simulink model "mod3_2plus1MASH_v2"  (Simulink 8.1)
settings: Solver=FixedStepDiscrete  StartTime=0.0  StopTime=80e-3  RelTol=1e-3
undefined symbols (not defined in the file): dfilt, Fs, modctrl
libraries: dspsigops x4, dspsrcs4 x2, dsparch4 x1
settings Model: Creator=amyles  LastModifiedBy=amyles
settings DataIOCC: MaxDataPoints=50000
settings OptimizationCC: InlineParams=on
settings DebuggingCC: StrictBusMsg=Warning
settings ModelReferenceCC: ModelReferenceNumInstancesAllowed=Single

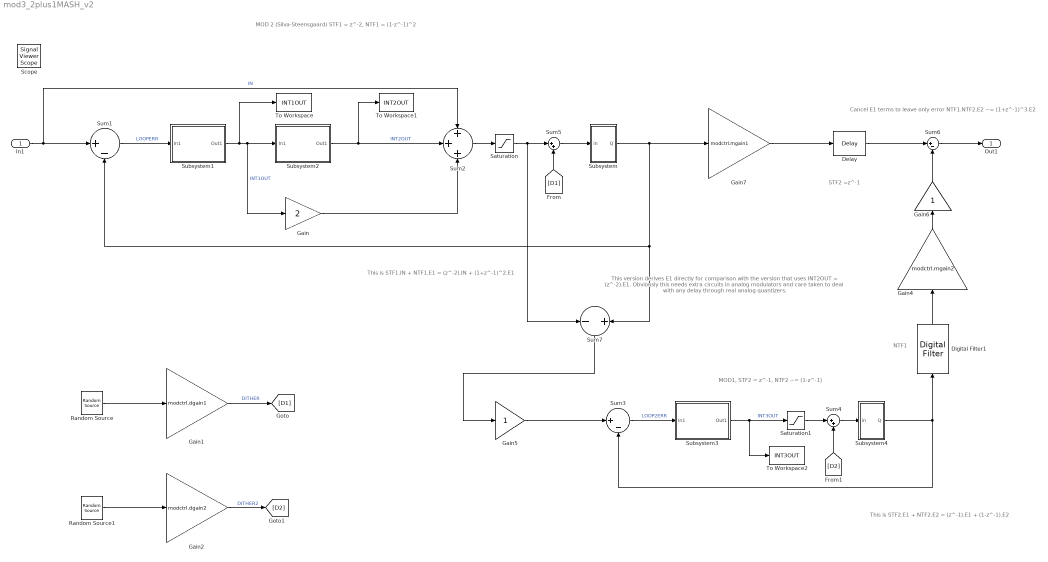
== system mod3_2plus1MASH_v2 ==
  note: MOD 2 (Silva-Steensgaard)
      | STF1 = z^-2, NTF1 = (1-z^-1)^2
  note: MOD1, STF2 = z^-1, NTF2 ~= (1-z^-1)
  note: This is STF2.E1 + NTF2.E2
      | = (z^-1).E1 + (1-z^-1).E2
  note: STF2
      | =z^-1
  note: NTF1
  note: Cancel E1 terms to leave
      | only error NTF1.NTF2.E2
      | ~= (1+z^-1)^3.E2
  note: This version derives E1
      | directly for comparison
      | with the version that uses
      | INT2OUT = (z^-2).E1.
      | Obviously this needs extra
      | circuits in analog modulators
      | and care taken to deal with
      | any delay through real
      | analog quantizers.
  note: This is STF1.IN + NTF1.E1
      | = (z^-2).IN + (1+z^-1)^2.E1
  In1 : Inport
  Delay : dspsigops/Delay  InputProcessing=Inherited (this choice will be removed - see release notes)  dly_unit=Samples  delay=1  ic_detail=off  dif_ic_for_ch=off  dif_ic_for_dly=off  ic=0  reset_popup=None
  Digital Filter1 : dsparch4/Digital Filter  TypePopup=FIR (all zeros)  IIRFiltStruct=Direct form II transposed  AllPoleFiltStruct=Direct form  FIRFiltStruct=Direct form  CoeffSource=Specify via dialog  NumCoeffs=[1 -2 1]  DenCoeffs=[1 0.1]  BiQuadCoeffs=[1 0.3 0.4 1 0.1 0.2]  LatticeCoeffs=[0.2 0.4]  denIgnore=on  FiltPerSampPopup=One filter per frame  IC=0  ICnum=0  ICden=0  roundingMode=Floor  overflowMode=off  ScaleValues=1  scaleValueFracLength=14  stageInFracLength=15  stageOutFracLength=15  FilterSource=Specify via dialog  dfiltObjectName=dfilt.dffir([1 2 1])  InputProcessing=Inherited (this choice will be removed - see release notes)
      settings: AttributesFormatString=NTF1 = (1-z^-1)^2
  Gain : Gain  Gain=2
  Gain1 : Gain  Gain=modctrl.dgain1
      settings: AttributesFormatString=Dither level adjust
  Gain2 : Gain  Gain=modctrl.dgain2
      settings: AttributesFormatString=Dither level adjust
  Gain4 : Gain  Gain=modctrl.mgain2
  Gain5 : Gain
      settings: AttributesFormatString=Option to scale input\nfor saturation control...
  Gain6 : Gain
      settings: AttributesFormatString=Option to un-scale input\npost saturation control...
  Gain7 : Gain  Gain=modctrl.mgain1
  Random Source : dspsrcs4/Random Source  SrcType=Uniform  NormMethod=Ziggurat  CltLength=12  MinVal=-1  MaxVal=1  MeanVal=0  VarVal=1  RepMode=Not repeatable  rawSeed=1  IsInherit=off  SampMode=Discrete  SampTime=1/Fs  SampFrame=1  DataType=Double  OutComplex=Real
      settings: AttributesFormatString=Dither source
  Random Source1 : dspsrcs4/Random Source  SrcType=Uniform  NormMethod=Ziggurat  CltLength=12  MinVal=-1  MaxVal=1  MeanVal=0  VarVal=1  RepMode=Not repeatable  rawSeed=1  IsInherit=off  SampMode=Discrete  SampTime=1/Fs  SampFrame=1  DataType=Double  OutComplex=Real
      settings: AttributesFormatString=Dither source
  Saturation : Saturate  UpperLimit=modctrl.qsatin1  LowerLimit=-(modctrl.qsatin1)
  Saturation1 : Saturate  UpperLimit=modctrl.qsatin2  LowerLimit=-(modctrl.qsatin2)
  Subsystem : Subsystem
      settings: AttributesFormatString=2-bit quantiser
  Subsystem1 : Subsystem
      settings: AttributesFormatString=Leaky delaying int
  Subsystem2 : Subsystem
      settings: AttributesFormatString=Leaky delaying int
  Subsystem3 : Subsystem
      settings: AttributesFormatString=Leaky delaying int
  Subsystem4 : Subsystem
      settings: AttributesFormatString=1-bit quantiser
  Sum1 : Sum  Inputs=|+-
      settings: AttributesFormatString=Modulator input\nloop servo error (input - fbk)
  Sum2 : Sum  Inputs=+++
  Sum3 : Sum  Inputs=|+-
      settings: AttributesFormatString=Modulator input\nloop servo error (input - fbk)
  Sum4 : Sum  Inputs=|++
  Sum5 : Sum  Inputs=|++
  Sum6 : Sum  Inputs=|+-
  Sum7 : Sum  Inputs=-|+
  To Workspace : ToWorkspace  VariableName=INT1OUT  SampleTime=-1
  To Workspace1 : ToWorkspace  VariableName=INT2OUT  SampleTime=-1
  To Workspace2 : ToWorkspace  VariableName=INT3OUT  SampleTime=-1
  Out1 : Outport
  Scope : SignalViewerScope  IOType=viewer  NumInputPorts=3  ZoomMode=xonly  RefreshTime=0.035000
      settings: YMin=-5~-5~-5  YMax=5~5~5
  wires:
  Sum1/1 -> Subsystem1/1(In1)  "LOOPERR"
  In1/1 -> Sum1/1, Sum2/1  "IN"
  Random Source/1 -> Gain1/1
  Gain/1 -> Sum2/3
  Sum5/1 -> Subsystem/1(in)
  Subsystem2/1(Out1) -> Sum2/2, To Workspace1/1  "INT2OUT"
  Sum3/1 -> Subsystem3/1(In1)  "LOOP2ERR"
  Subsystem1/1(Out1) -> Subsystem2/1(In1), Gain/1, To Workspace/1  "INT1OUT"
  Sum2/1 -> Saturation/1
  Subsystem3/1(Out1) -> Saturation1/1, To Workspace2/1  "INT3OUT"
  Sum4/1 -> Subsystem4/1(in)
  Subsystem4/1(Q) -> Sum3/2, Digital Filter1/1
  Random Source1/1 -> Gain2/1
  Delay/1 -> Sum6/1
  Gain4/1 -> Gain6/1
  Sum6/1 -> Out1/1
  Digital Filter1/1 -> Gain4/1
  Gain5/1 -> Sum3/1
  Gain6/1 -> Sum6/2
  Subsystem/1(Q) -> Sum1/2, Sum7/2, Gain7/1
  Gain1/1 -> [D1]  "DITHER"
  Gain2/1 -> [D2]  "DITHER2"
  [D1] -> Sum5/2
  [D2] -> Sum4/2
  Saturation/1 -> Sum5/1, Sum7/1
  Saturation1/1 -> Sum4/1
  Sum7/1 -> Gain5/1
  Gain7/1 -> Delay/1

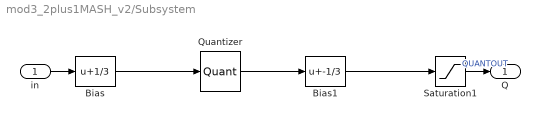
== system mod3_2plus1MASH_v2/Subsystem ==
  in : Inport
  Bias : Bias  Bias=1/3
      settings: AttributesFormatString=Need offset to give\nMID-RISE quantiser
  Bias1 : Bias  Bias=-1/3
  Quantizer : Quantizer  QuantizationInterval=2/3  LinearizeAsGain=off
  Saturation1 : Saturate  UpperLimit=1  LowerLimit=-1
      settings: AttributesFormatString=Limit quantiser\noutput to +/-1
  Q : Outport
  wires:
  Bias/1 -> Quantizer/1
  Quantizer/1 -> Bias1/1
  Bias1/1 -> Saturation1/1
  in/1 -> Bias/1
  Saturation1/1 -> Q/1  "QUANTOUT"

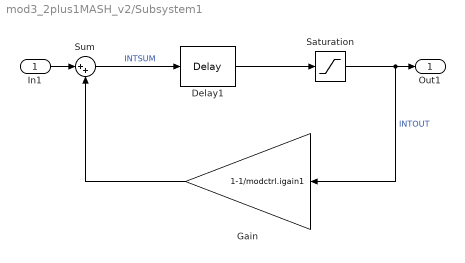
== system mod3_2plus1MASH_v2/Subsystem1 ==
  In1 : Inport
  Delay1 : dspsigops/Delay  dly_unit=Samples  delay=1  ic_detail=off  dif_ic_for_ch=off  dif_ic_for_dly=off  ic=0  reset_popup=None
  Gain : Gain  Gain=1-1/modctrl.igain1
      settings: AttributesFormatString=Integrator leakage
  Saturation : Saturate  UpperLimit=modctrl.isat1  LowerLimit=-(modctrl.isat1)
  Sum : Sum  Inputs=|++
      settings: AttributesFormatString=Integrator summer
  Out1 : Outport
  wires:
  Sum/1 -> Delay1/1  "INTSUM"
  Gain/1 -> Sum/2
  Saturation/1 -> Gain/1, Out1/1  "INTOUT"
  Delay1/1 -> Saturation/1
  In1/1 -> Sum/1

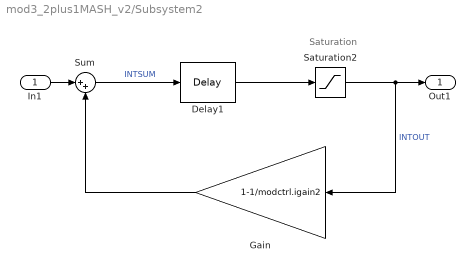
== system mod3_2plus1MASH_v2/Subsystem2 ==
  note: Saturation
  In1 : Inport
  Delay1 : dspsigops/Delay  dly_unit=Samples  delay=1  ic_detail=off  dif_ic_for_ch=off  dif_ic_for_dly=off  ic=0  reset_popup=None
  Gain : Gain  Gain=1-1/modctrl.igain2
      settings: AttributesFormatString=Integrator leakage
  Saturation2 : Saturate  UpperLimit=modctrl.isat2  LowerLimit=-(modctrl.isat2)
  Sum : Sum  Inputs=|++
      settings: AttributesFormatString=Integrator summer
  Out1 : Outport
  wires:
  In1/1 -> Sum/1
  Delay1/1 -> Saturation2/1
  Saturation2/1 -> Out1/1, Gain/1  "INTOUT"
  Gain/1 -> Sum/2
  Sum/1 -> Delay1/1  "INTSUM"

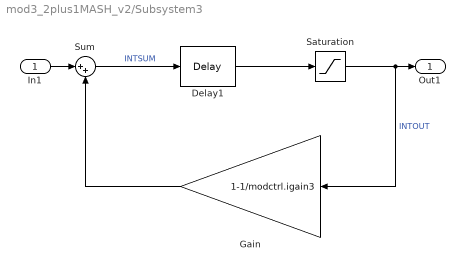
== system mod3_2plus1MASH_v2/Subsystem3 ==
  In1 : Inport
  Delay1 : dspsigops/Delay  dly_unit=Samples  delay=1  ic_detail=off  dif_ic_for_ch=off  dif_ic_for_dly=off  ic=0  reset_popup=None
  Gain : Gain  Gain=1-1/modctrl.igain3
      settings: AttributesFormatString=Integrator leakage
  Saturation : Saturate  UpperLimit=modctrl.isat3  LowerLimit=-(modctrl.isat3)
  Sum : Sum  Inputs=|++
      settings: AttributesFormatString=Integrator summer
  Out1 : Outport
  wires:
  In1/1 -> Sum/1
  Delay1/1 -> Saturation/1
  Saturation/1 -> Out1/1, Gain/1  "INTOUT"
  Gain/1 -> Sum/2
  Sum/1 -> Delay1/1  "INTSUM"

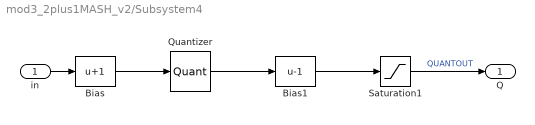
== system mod3_2plus1MASH_v2/Subsystem4 ==
  in : Inport
  Bias : Bias  Bias=1
      settings: AttributesFormatString=Need offset to give\nMID-RISE quantiser
  Bias1 : Bias  Bias=-1
      settings: AttributesFormatString=1
  Quantizer : Quantizer  QuantizationInterval=2  LinearizeAsGain=off
  Saturation1 : Saturate  UpperLimit=1  LowerLimit=-1
      settings: AttributesFormatString=Limit quantiser\noutput to +/-1
  Q : Outport
  wires:
  Saturation1/1 -> Q/1  "QUANTOUT"
  in/1 -> Bias/1
  Bias1/1 -> Saturation1/1
  Quantizer/1 -> Bias1/1
  Bias/1 -> Quantizer/1
